simulink model "TwoRegion_swing_NotSoFineTimeStep"  (R2017b)
settings: Solver=FixedStepAuto  StartTime=0.0  StopTime=10  FixedStep=0.001  RelTol=1e-3  EnableMultiTasking=on
values from neighbouring files (symbols this model uses):
  D = [0.5e-2 0.5e-2]    [Energy_nadir_analysis.m]
  H1 = fraction_H*H    [Energy_nadir_analysis.m]
  H2 = (1-fraction_H)*H    [Energy_nadir_analysis.m]
  P_D = Demand*[fraction_D (1-fraction_D)]    [Energy_nadir_analysis.m]
  PFR1 = fraction_R*R    [Energy_nadir_analysis.m]
  PFR2 = (1-fraction_R)*R    [Energy_nadir_analysis.m]
  Td = 10    [Energy_nadir_analysis.m]
  V = 345    [Energy_nadir_analysis.m]
  X = 50    [Energy_nadir_analysis.m]
undefined symbols (not defined in the file or in its folder): P_loss
libraries: simulink x2
settings Model: Creator=lb2916  LastModifiedBy=Luis
settings OptimizationCC: LifeSpan=inf
settings DebuggingCC: SFUnexpectedBacktrackingDiag=warning  SFNoUnconditionalDefaultTransitionDiag=warning  SFExecutionAtInitializationDiag=none
settings CodeAppCC: StateflowObjectComments=on
settings GRTTargetCC: TargetLangStandard=C89/C90 (ANSI)  GeneratePreprocessorConditionals=Disable all
settings ConfigComp: CovMetricSettings=dw  CovHtmlReporting=on  CovSaveCumulativeToWorkspaceVar=on  CovSaveSingleToWorkspaceVar=on  CovExternalEMLEnable=off

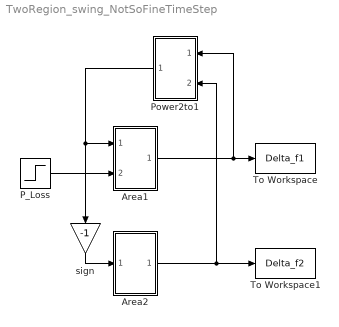
== system TwoRegion_swing_NotSoFineTimeStep ==
  Area1 : Subsystem
  Area2 : Subsystem
  P_Loss : Step  Time=1000  Before=P_loss  After=P_loss  SampleTime=0
  Power2to1 : Subsystem
  To Workspace : ToWorkspace  VariableName=Delta_f1  SaveFormat=Timeseries  SampleTime=-1
  To Workspace1 : ToWorkspace  VariableName=Delta_f2  SaveFormat=Timeseries  SampleTime=-1
  sign : Gain  Gain=-1
  wires:
  Area1/1(Out1) -> To Workspace/1, Power2to1/1(In1)
  P_Loss/1 -> Area1/2(In2)
  Area2/1(Out1) -> Power2to1/2(In2), To Workspace1/1
  Power2to1/1(Out1) -> Area1/1(In1), sign/1
  sign/1 -> Area2/1(In1)

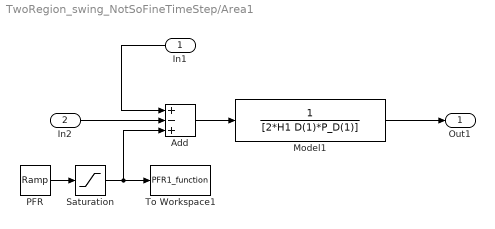
== system TwoRegion_swing_NotSoFineTimeStep/Area1 ==
  In1 : Inport
  In2 : Inport  Port=2
  Add : Sum  Inputs=+-+
  Model1 : TransferFcn  Denominator=[2*H1 D(1)*P_D(1)]
  PFR : simulink/Sources/Ramp  slope=PFR1/Td  start=0  X0=0
  Saturation : Saturate  UpperLimit=PFR1  LowerLimit=0
  To Workspace1 : ToWorkspace  VariableName=PFR1_function  SaveFormat=Timeseries  SampleTime=-1
  Out1 : Outport
  wires:
  In2/1 -> Add/2
  Model1/1 -> Out1/1
  Add/1 -> Model1/1
  In1/1 -> Add/1
  Saturation/1 -> Add/3, To Workspace1/1
  PFR/1 -> Saturation/1

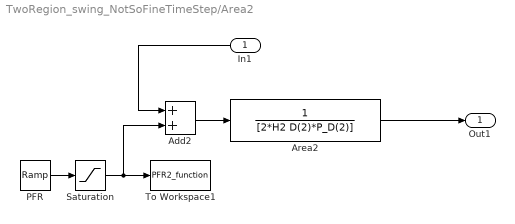
== system TwoRegion_swing_NotSoFineTimeStep/Area2 ==
  In1 : Inport
  Add2 : Sum
  Area2 : TransferFcn  Denominator=[2*H2 D(2)*P_D(2)]
  PFR : simulink/Sources/Ramp  slope=PFR2/Td  start=0  X0=0
  Saturation : Saturate  UpperLimit=PFR2  LowerLimit=0
  To Workspace1 : ToWorkspace  VariableName=PFR2_function  SaveFormat=Timeseries  SampleTime=-1
  Out1 : Outport
  wires:
  Area2/1 -> Out1/1
  Add2/1 -> Area2/1
  In1/1 -> Add2/1
  Saturation/1 -> Add2/2, To Workspace1/1
  PFR/1 -> Saturation/1

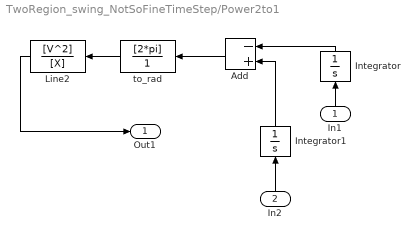
== system TwoRegion_swing_NotSoFineTimeStep/Power2to1 ==
  In1 : Inport
  In2 : Inport  Port=2
  Add : Sum  Inputs=-+
  Integrator : Integrator
  Integrator1 : Integrator
  Line2 : TransferFcn  Numerator=[V^2]  Denominator=[X]
  to_rad : TransferFcn  Numerator=[2*pi]  Denominator=[1]
  Out1 : Outport
  wires:
  Line2/1 -> Out1/1
  Add/1 -> to_rad/1
  to_rad/1 -> Line2/1
  In1/1 -> Integrator/1
  Integrator/1 -> Add/1
  In2/1 -> Integrator1/1
  Integrator1/1 -> Add/2
